simulink model "filters_example"  (R2015b)
settings: Solver=VariableStepAuto  StartTime=0.0  StopTime=20  RelTol=1e-3
values from neighbouring files (symbols this model uses):
  KF_R = diag([0.1,0.1,0.1,0.01,0.01,0.01,0.0001,0.0001,0.0001])    [init_filters_example.m]
undefined symbols (not defined in the file or in its folder): Do, euleranglelim, innerLoopSampleRate, Io, KF_C, N, omegalim, Po, seed
libraries: simulink x2, vrlib x2
settings Model: Creator=Daniel  LastModifiedBy=mgreiff
settings SolverCC: AlgebraicLoopSolver=LineSearch

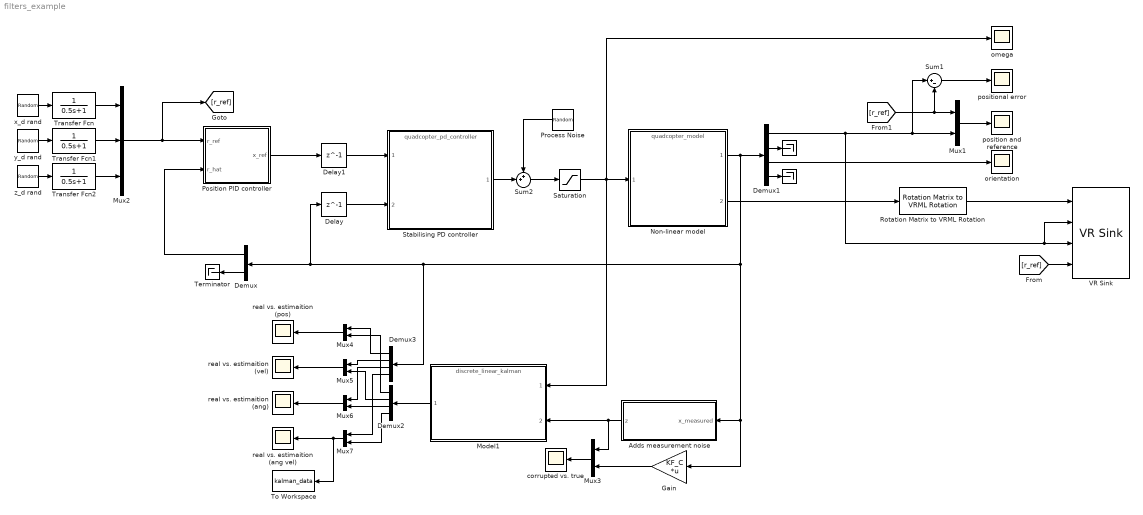
== system filters_example ==
  "  " : Terminator
  "   " : Terminator
  Adds measurement noise : Subsystem
  Delay : Delay  DelayLength=1  InitialCondition=0  SampleTime=innerLoopSampleRate
  Delay1 : Delay  DelayLength=1  InitialCondition=0  SampleTime=innerLoopSampleRate
  Demux : Demux  Outputs=[3,9]
  Demux1 : Demux  Outputs=[3,3,3,3]
  Demux2 : Demux  Outputs=[3,3,3,3]
  Demux3 : Demux  Outputs=[3,3,3,3]
  Gain : Gain  Gain=KF_C  Multiplication=Matrix(K*u)
  Model1 : ModelReference  ModelNameDialog=discrete_linear_kalman.slx  SimulationMode=Normal  ModelReferenceVersion=1.88  CopyOfModelName=discrete_linear_kalman.slx
  Mux{1,3..7} (6 alike) : Mux  Inputs=2
  Mux2 : Mux  Inputs=3
  Non-linear model : ModelReference  ModelNameDialog=quadcopter_model.mdl  SimulationMode=Normal  ModelReferenceVersion=1.117  CopyOfModelName=quadcopter_model.mdl
  Position PID controller : Subsystem
  Process Noise : RandomNumber  Mean=[0 0 0 0]'  Variance=0  SampleTime=0.5
  Rotation Matrix to VRML Rotation : vrlib/Utilities/Rotation Matrix to VRML Rotation  maxzero=1e-12
  Saturation : Saturate  UpperLimit=omegalim(2)  LowerLimit=omegalim(1)
  Stabilising PD controller : ModelReference  ModelNameDialog=quadcopter_pd_controller.mdl  SimulationMode=Normal  ModelReferenceVersion=1.68  CopyOfModelName=quadcopter_pd_controller.mdl
  Sum1 : Sum  Inputs=|+-
  Sum2 : Sum  Inputs=++|
  Terminator : Terminator
  To Workspace : ToWorkspace  VariableName=kalman_data  SaveFormat=Timeseries  SampleTime=-1
  Transfer Fcn : TransferFcn  Denominator=[0.5 1]
  Transfer Fcn1 : TransferFcn  Denominator=[0.5 1]
  Transfer Fcn2 : TransferFcn  Denominator=[0.5 1]
  VR Sink : vrlib/VR Sink  InstantiateOnLoad=on  SampleTime=0.05  ViewEnable=on  RemoteChange=off  RemoteView=off  FieldsWritten=copter.rotation.4.1.1.double#copter.translation.3.1.1.double#vp.translation.3.1.1.double#target.translation.3.1.1.double  WorldFileName=copter_world.wrl  WorldDescription=quadcopter_world  AutoView=on  VideoDimensions=[]  AllowVariableSize=off
  corrupted vs. true : Scope
  "omega " : Scope
  orientation : Scope
  position and reference : Scope
  positional error : Scope
  real vs. estimaition (ang vel) : Scope
  real vs. estimaition (ang) : Scope
  real vs. estimaition (pos) : Scope
  real vs. estimaition (vel) : Scope
  x_d rand : UniformRandomNumber  Minimum=-30  Maximum=30  Seed=0+seed  SampleTime=10
  y_d rand : UniformRandomNumber  Minimum=-30  Maximum=30  Seed=1+seed  SampleTime=10
  z_d rand : UniformRandomNumber  Minimum=0  Maximum=15  Seed=2+seed  SampleTime=10
  wires:
  Non-linear model/2 -> Rotation Matrix to VRML Rotation/1
  x_d rand/1 -> Transfer Fcn/1
  y_d rand/1 -> Transfer Fcn1/1
  z_d rand/1 -> Transfer Fcn2/1
  Rotation Matrix to VRML Rotation/1 -> VR Sink/1
  Mux2/1 -> [r_ref], Position PID controller/1(r_ref)
  Transfer Fcn/1 -> Mux2/1
  Transfer Fcn1/1 -> Mux2/2
  Transfer Fcn2/1 -> Mux2/3
  Process Noise/1 -> Sum2/1
  Sum2/1 -> Saturation/1
  Saturation/1 -> Model1/1, "omega "/1, Non-linear model/1
  Stabilising PD controller/1 -> Sum2/2
  Position PID controller/1(x_ref) -> Delay1/1
  Non-linear model/1 -> Delay/1, Demux/1, Demux3/1, Adds measurement noise/1(x_measured), Gain/1, Demux1/1
  Demux/2 -> Terminator/1
  Demux/1 -> Position PID controller/2(r_hat)
  [r_ref] -> VR Sink/4
  [r_ref] -> Sum1/2, Mux1/1
  Mux1/1 -> position and reference/1
  Sum1/1 -> positional error/1
  Demux1/1 -> VR Sink/2, VR Sink/3, Sum1/1, Mux1/2
  Demux1/2 -> "  "/1
  Demux1/4 -> "   "/1
  Demux1/3 -> orientation/1
  Adds measurement noise/1(z) -> Model1/2, Mux3/1
  Gain/1 -> Mux3/2
  Mux3/1 -> corrupted vs. true/1
  Model1/1 -> Demux2/1
  Mux4/1 -> real vs. estimaition (pos)/1
  Mux5/1 -> real vs. estimaition (vel)/1
  Mux6/1 -> real vs. estimaition (ang)/1
  Mux7/1 -> To Workspace/1, real vs. estimaition (ang vel)/1
  Demux3/1 -> Mux4/1
  Demux2/1 -> Mux4/2
  Demux3/2 -> Mux5/1
  Demux2/2 -> Mux5/2
  Demux3/3 -> Mux6/1
  Demux2/3 -> Mux6/2
  Demux2/4 -> Mux7/2
  Demux3/4 -> Mux7/1
  Delay/1 -> Stabilising PD controller/2
  Delay1/1 -> Stabilising PD controller/1

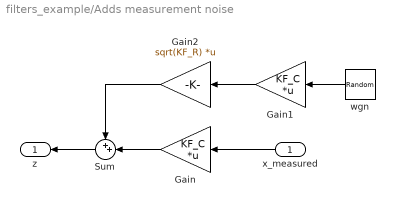
== system filters_example/Adds measurement noise ==
  x_measured : Inport
  Gain : Gain  Gain=KF_C  Multiplication=Matrix(K*u)
  Gain1 : Gain  Gain=KF_C  Multiplication=Matrix(K*u)
  Gain2 : Gain  Gain=sqrt(KF_R)  Multiplication=Matrix(K*u)
  Sum : Sum  Inputs=++|
  wgn : RandomNumber  Mean=[0 0 0 0 0 0 0 0 0 0 0 0]'
  z : Outport
  wires:
  x_measured/1 -> Gain/1
  Gain1/1 -> Gain2/1
  Sum/1 -> z/1
  Gain/1 -> Sum/2
  Gain2/1 -> Sum/1
  wgn/1 -> Gain1/1

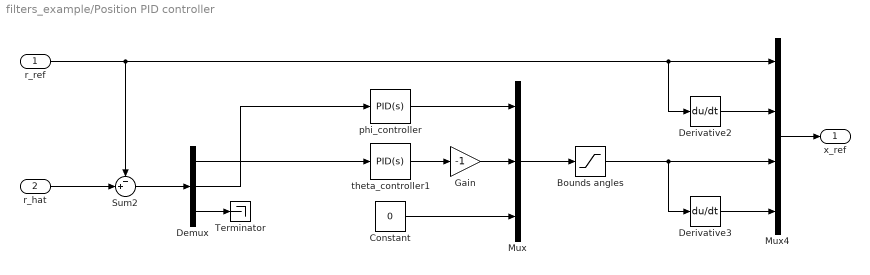
== system filters_example/Position PID controller ==
  r_ref : Inport
  r_hat : Inport  Port=2
  Bounds angles : Saturate  UpperLimit=euleranglelim(2)  LowerLimit=euleranglelim(1)
  Constant : Constant  Value=0
  Demux : Demux  Outputs=3
  Derivative2 : Derivative
  Derivative3 : Derivative
  Gain : Gain  Gain=-1
  Mux : Mux  Inputs=3
  Mux4 : Mux  Inputs=[3,3,3,3]
  Sum2 : Sum  Inputs=-+|
  Terminator : Terminator
  phi_controller : simulink/Continuous/PID Controller  Controller=PID  TimeDomain=Continuous-time  SampleTime=-1  IntegratorMethod=Forward Euler  FilterMethod=Forward Euler  Form=Parallel  UseFilter=on  ControllerParametersSource=internal  P=Po  I=Io  D=Do  N=N  InitialConditionSource=internal  InitialConditionForIntegrator=0  InitialConditionForFilter=0  ExternalReset=none  LimitOutput=off  UpperSaturationLimit=inf  LowerSaturationLimit=-inf  LinearizeAsGain=on  AntiWindupMode=none  Kb=1  TrackingMode=off  Kt=1  PParamMin=[]  PParamMax=[]  IParamMin=[]  IParamMax=[]  DParamMin=[]  DParamMax=[]  NParamMin=[]  NParamMax=[]  KbParamMin=[]  KbParamMax=[]  KtParamMin=[]  KtParamMax=[]  POutMin=[]  POutMax=[]  IOutMin=[]  IOutMax=[]  DOutMin=[]  DOutMax=[]  NOutMin=[]  NOutMax=[]  KbOutMin=[]  KbOutMax=[]  KtOutMin=[]  KtOutMax=[]  IntegratorOutMin=[]  IntegratorOutMax=[]  FilterOutMin=[]  FilterOutMax=[]  SumOutMin=[]  SumOutMax=[]  SumI1OutMin=[]  SumI1OutMax=[]  SumI2OutMin=[]  SumI2OutMax=[]  SumI3OutMin=[]  SumI3OutMax=[]  SumDOutMin=[]  SumDOutMax=[]  SaturationOutMin=[]  SaturationOutMax=[]  IntegratorContinuousStateAttributes=''  IntegratorStateMustResolveToSignalObject=off  IntegratorRTWStateStorageClass=Auto  FilterContinuousStateAttributes=''  FilterStateMustResolveToSignalObject=off  FilterRTWStateStorageClass=Auto  DifferentiatorICPrevScaledInput=0  DifferentiatorOutMin=[]  DifferentiatorOutMax=[]
  theta_controller1 : simulink/Continuous/PID Controller  Controller=PID  TimeDomain=Continuous-time  SampleTime=-1  IntegratorMethod=Forward Euler  FilterMethod=Forward Euler  Form=Parallel  UseFilter=on  ControllerParametersSource=internal  P=Po  I=Io  D=Do  N=N  InitialConditionSource=internal  InitialConditionForIntegrator=0  InitialConditionForFilter=0  ExternalReset=none  LimitOutput=off  UpperSaturationLimit=inf  LowerSaturationLimit=-inf  LinearizeAsGain=on  AntiWindupMode=none  Kb=1  TrackingMode=off  Kt=1  PParamMin=[]  PParamMax=[]  IParamMin=[]  IParamMax=[]  DParamMin=[]  DParamMax=[]  NParamMin=[]  NParamMax=[]  KbParamMin=[]  KbParamMax=[]  KtParamMin=[]  KtParamMax=[]  POutMin=[]  POutMax=[]  IOutMin=[]  IOutMax=[]  DOutMin=[]  DOutMax=[]  NOutMin=[]  NOutMax=[]  KbOutMin=[]  KbOutMax=[]  KtOutMin=[]  KtOutMax=[]  IntegratorOutMin=[]  IntegratorOutMax=[]  FilterOutMin=[]  FilterOutMax=[]  SumOutMin=[]  SumOutMax=[]  SumI1OutMin=[]  SumI1OutMax=[]  SumI2OutMin=[]  SumI2OutMax=[]  SumI3OutMin=[]  SumI3OutMax=[]  SumDOutMin=[]  SumDOutMax=[]  SaturationOutMin=[]  SaturationOutMax=[]  IntegratorContinuousStateAttributes=''  IntegratorStateMustResolveToSignalObject=off  IntegratorRTWStateStorageClass=Auto  FilterContinuousStateAttributes=''  FilterStateMustResolveToSignalObject=off  FilterRTWStateStorageClass=Auto  DifferentiatorICPrevScaledInput=0  DifferentiatorOutMin=[]  DifferentiatorOutMax=[]
  x_ref : Outport
  wires:
  Constant/1 -> Mux/3
  theta_controller1/1 -> Gain/1
  phi_controller/1 -> Mux/1
  Demux/3 -> Terminator/1
  Demux/1 -> theta_controller1/1
  Demux/2 -> phi_controller/1
  Gain/1 -> Mux/2
  Mux/1 -> Bounds angles/1
  r_hat/1 -> Sum2/2
  Sum2/1 -> Demux/1
  Bounds angles/1 -> Derivative3/1, Mux4/3
  r_ref/1 -> Sum2/1, Derivative2/1, Mux4/1
  Derivative2/1 -> Mux4/2
  Derivative3/1 -> Mux4/4
  Mux4/1 -> x_ref/1
